simulink model "maglev_sim"  (R2022a)
settings: Solver=VariableStepAuto  StartTime=0.0  StopTime=5  RelTol=1e-3
values from neighbouring files (symbols this model uses):
  A = [ ... (first row only)    [hw3.m]    (also in maglev.m = raw_A - B*K_leader)
  Adj = full(adjacency(Gr))    [hw3.m]    (also in maglev.m = full(adjacency(Gr, 'weighted')))
  B = [0; 1/m1; 0; 0]    [hw3.m]    (also in maglev.m = [0; -9.9453])
  c = 0.7    [hw3.m]    (also in maglev.m = c_values(i))
  C = eye(4)    [hw3.m]    (also in maglev.m = [708.27 0])
  D = diag(in_degrees)    [hw3.m]    (also in maglev.m = 0)
  F = zeros(size(F))    [maglev.m]
  K = inv(R)*(B')*P    [hw3.m]    (also in maglev.m)
  K_leader = acker(raw_A, B, poles)    [maglev.m]
  pins = [1 0 0 0 0 0]    [hw3.m]    (also in maglev.m)
libraries: eeLuenbergerObserver x5
settings Model: Creator=jules  LastModifiedBy=jules
settings DebuggingCC: AllowedUnitSystems=SI,SI (extended)

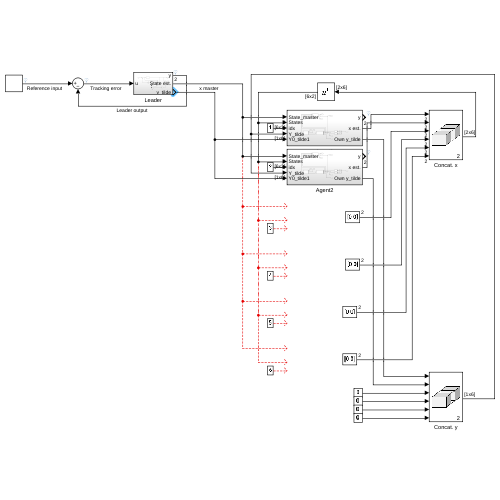
[thumbnail: Simulink's stored preview of the top-level diagram]
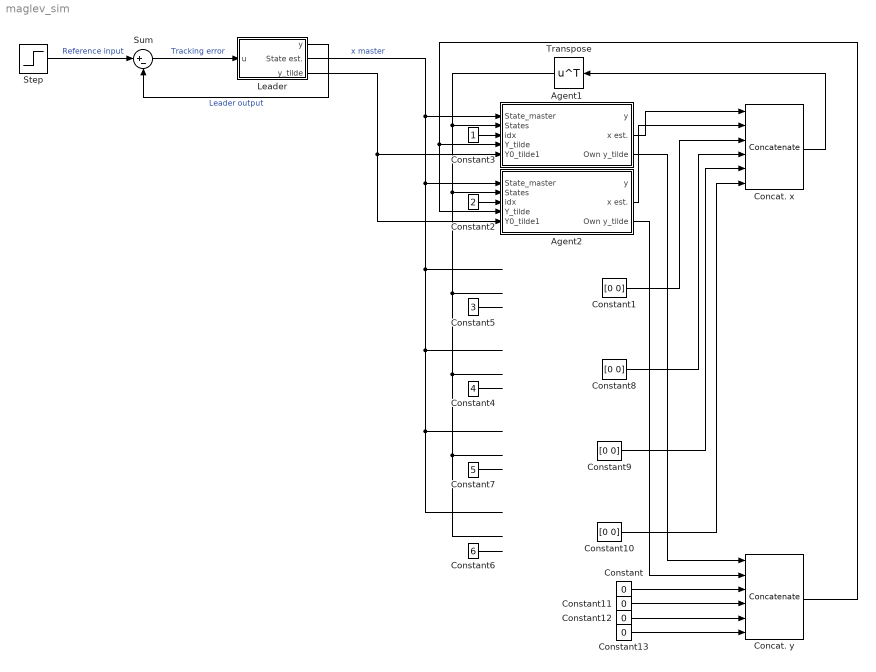
== system maglev_sim ==
  Agent1 : Subsystem
  Agent2 : Subsystem
  Concat. x : Concatenate  NumInputs=6  Mode=Multidimensional array  ConcatenateDimension=2
  Concat. y : Concatenate  NumInputs=6  Mode=Multidimensional array  ConcatenateDimension=2
  Constant{,11..13} (4 alike) : Constant  Value=0
  Constant{1,8..10} (4 alike) : Constant  Value=[0 0]
  Constant2 : Constant  Value=2
  Constant3 : Constant
  Constant4 : Constant  Value=4
  Constant5 : Constant  Value=3
  Constant6 : Constant  Value=6
  Constant7 : Constant  Value=5
  Leader : Subsystem
  Step : Step  SampleTime=0
  Sum : Sum  Inputs=|+-
  Transpose : Math  Operator=transpose
  wires:
  Leader/2(State est.) -> Agent2/1(State_master), Agent1/1(State_master)  "x master"
  Constant3/1 -> Agent1/3(idx)
  Constant4/1 -> ?
  Constant5/1 -> ?
  Constant6/1 -> ?
  Constant7/1 -> ?
  Concat. x/1 -> Transpose/1
  Constant1/1 -> Concat. x/3
  Constant8/1 -> Concat. x/4
  Constant9/1 -> Concat. x/5
  Constant10/1 -> Concat. x/6
  Transpose/1 -> Agent2/2(States), Agent1/2(States)
  Step/1 -> Sum/1  "Reference input"
  Sum/1 -> Leader/1(u)  "Tracking error"
  Leader/1(y) -> Sum/2  "Leader output"
  Agent1/2(x est.) -> Concat. x/1
  Agent1/3(Own y_tilde) -> Concat. y/1
  Constant13/1 -> Concat. y/6
  Constant12/1 -> Concat. y/5
  Constant11/1 -> Concat. y/4
  Constant/1 -> Concat. y/3
  Concat. y/1 -> Agent1/4(Y_tilde), Agent2/4(Y_tilde)
  Constant2/1 -> Agent2/3(idx)
  Agent2/2(x est.) -> Concat. x/2
  Agent2/3(Own y_tilde) -> Concat. y/2
  Leader/3(y_tilde) -> Agent1/5(Y0_tilde1), Agent2/5(Y0_tilde1)

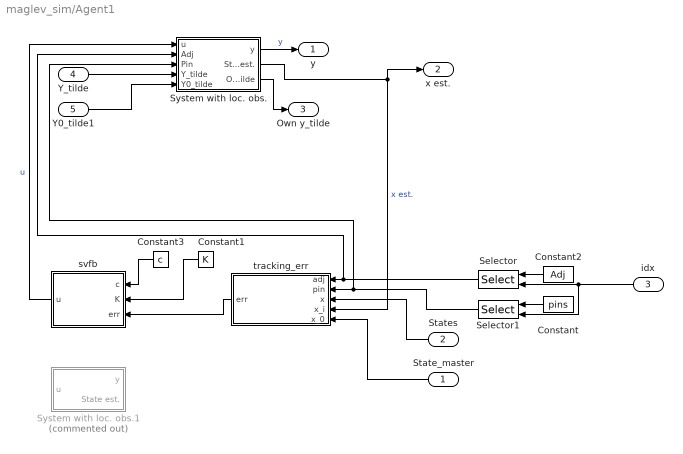
== system maglev_sim/Agent1 ==
  State_master : Inport
  States : Inport  Port=2
  idx : Inport  Port=3
  Y_tilde : Inport  Port=4
  Y0_tilde1 : Inport  Port=5
  Constant : Constant  Value=pins
  Constant1 : Constant  Value=K  VectorParams1D=off
  Constant2 : Constant  Value=Adj  VectorParams1D=off
  Constant3 : Constant  Value=c
  Selector : Selector  NumberOfDimensions=2  InputPortWidth=[6 6]  IndexOptions=Select all,Index vector (port)  Indices=[1 3],1  OutputSizes=1,1
  Selector1 : Selector  InputPortWidth=6  IndexOptions=Index vector (port)  Indices=[1 3]  OutputSizes=1
  System with loc. obs. : Subsystem
  System with loc. obs.1 : Subsystem  Commented=on
  svfb : MATLAB Function  TreatAsAtomicUnit=on
  tracking_err : MATLAB Function  TreatAsAtomicUnit=on
  y : Outport
  x est. : Outport  Port=2
  Own y_tilde : Outport  Port=3
  wires:
  idx/1 -> Selector1/2, Selector/2
  Constant2/1 -> Selector/1
  System with loc. obs./1(y) -> y/1  "y"
  svfb/1(u) -> System with loc. obs./1(u)  "u"
  System with loc. obs./2(State est.) -> tracking_err/4(x_i), x est./1  "x est."
  tracking_err/1(err) -> svfb/3(err)
  Constant/1 -> Selector1/1
  Constant1/1 -> svfb/2(K)
  Constant3/1 -> svfb/1(c)
  States/1 -> tracking_err/3(x)
  State_master/1 -> tracking_err/5(x_0)
  Selector1/1 -> tracking_err/2(pin), System with loc. obs./3(Pin)
  Selector/1 -> System with loc. obs./2(Adj), tracking_err/1(adj)
  System with loc. obs./3(Own y_tilde) -> Own y_tilde/1
  Y_tilde/1 -> System with loc. obs./4(Y_tilde)
  Y0_tilde1/1 -> System with loc. obs./5(Y0_tilde)

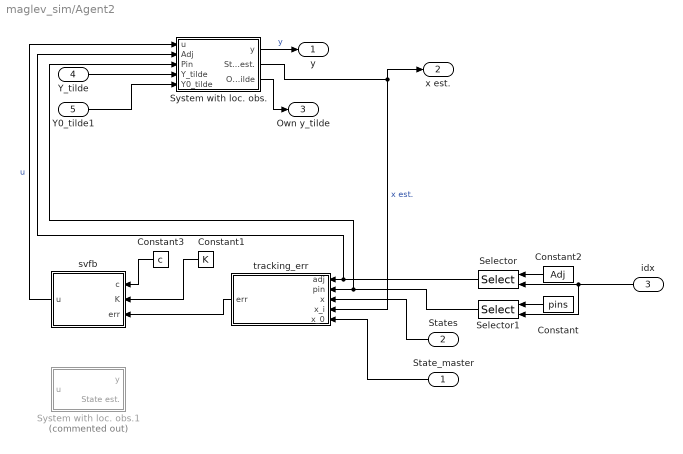
== system maglev_sim/Agent2 ==
  State_master : Inport
  States : Inport  Port=2
  idx : Inport  Port=3
  Y_tilde : Inport  Port=4
  Y0_tilde1 : Inport  Port=5
  Constant : Constant  Value=pins
  Constant1 : Constant  Value=K  VectorParams1D=off
  Constant2 : Constant  Value=Adj  VectorParams1D=off
  Constant3 : Constant  Value=c
  Selector : Selector  NumberOfDimensions=2  InputPortWidth=[6 6]  IndexOptions=Select all,Index vector (port)  Indices=[1 3],1  OutputSizes=1,1
  Selector1 : Selector  InputPortWidth=6  IndexOptions=Index vector (port)  Indices=[1 3]  OutputSizes=1
  System with loc. obs. : Subsystem
  System with loc. obs.1 : Subsystem  Commented=on
  svfb : MATLAB Function  TreatAsAtomicUnit=on
  tracking_err : MATLAB Function  TreatAsAtomicUnit=on
  y : Outport
  x est. : Outport  Port=2
  Own y_tilde : Outport  Port=3
  wires:
  idx/1 -> Selector1/2, Selector/2
  Constant2/1 -> Selector/1
  System with loc. obs./1(y) -> y/1  "y"
  svfb/1(u) -> System with loc. obs./1(u)  "u"
  System with loc. obs./2(State est.) -> tracking_err/4(x_i), x est./1  "x est."
  tracking_err/1(err) -> svfb/3(err)
  Constant/1 -> Selector1/1
  Constant1/1 -> svfb/2(K)
  Constant3/1 -> svfb/1(c)
  States/1 -> tracking_err/3(x)
  State_master/1 -> tracking_err/5(x_0)
  Selector1/1 -> tracking_err/2(pin), System with loc. obs./3(Pin)
  Selector/1 -> System with loc. obs./2(Adj), tracking_err/1(adj)
  System with loc. obs./3(Own y_tilde) -> Own y_tilde/1
  Y_tilde/1 -> System with loc. obs./4(Y_tilde)
  Y0_tilde1/1 -> System with loc. obs./5(Y0_tilde)

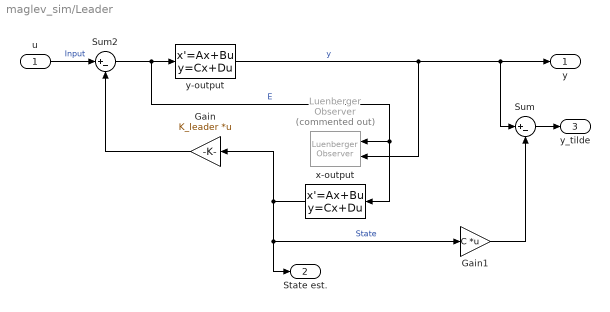
== system maglev_sim/Leader ==
  u : Inport
  Gain : Gain  Gain=K_leader  Multiplication=Matrix(K*u)
  Gain1 : Gain  Gain=C  Multiplication=Matrix(K*u)
  Luenberger Observer : eeLuenbergerObserver/Luenberger Observer  Commented=on  StateSpaceType=Continuous-time  Ad=A  Bd=1  Cd=1  Dd=1  A=A  B=B  C=C  D=[0]  ObserverDesign=Desired eigenvalues  Ld=1  DesiredEigenvalues=[-10 -20]  x0=[0 0]  Tsd=0.1  Ts=0.1
      settings: SourceProductBaseCode=PS
  Sum : Sum  Inputs=|+-
  Sum2 : Sum  Inputs=|+-
  x-output : StateSpace  A=A  B=B  C=eye(2)  D=[0; 0]  InitialCondition=0
  y-output : StateSpace  A=A  B=B  C=C  D=D  InitialCondition=0
  y : Outport
  State est. : Outport  Port=2
  y_tilde : Outport  Port=3
  wires:
  Gain/1 -> Sum2/2
  y-output/1 -> Luenberger Observer/2, Sum/1, y/1  "y"
  u/1 -> Sum2/1  "Input"
  Sum2/1 -> Luenberger Observer/1, x-output/1, y-output/1  "E"
  x-output/1 -> Gain1/1, State est./1, Gain/1  "State"
  Gain1/1 -> Sum/2
  Sum/1 -> y_tilde/1

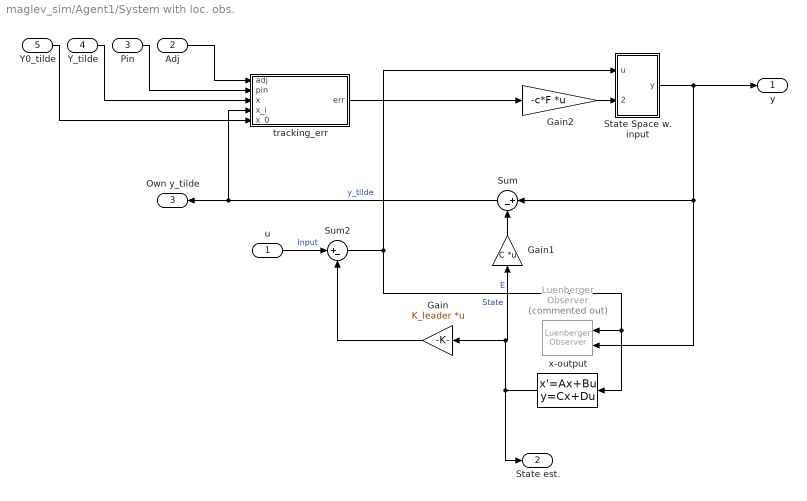
== system maglev_sim/Agent1/System with loc. obs. ==
  u : Inport
  Adj : Inport  Port=2
  Pin : Inport  Port=3
  Y_tilde : Inport  Port=4
  Y0_tilde : Inport  Port=5
  Gain : Gain  Gain=K_leader  Multiplication=Matrix(K*u)
  Gain1 : Gain  Gain=C  Multiplication=Matrix(K*u)
  Gain2 : Gain  Gain=-c*F  Multiplication=Matrix(K*u)
  Luenberger Observer : eeLuenbergerObserver/Luenberger Observer  Commented=on  StateSpaceType=Continuous-time  Ad=A  Bd=1  Cd=1  Dd=1  A=A  B=B  C=C  D=[0]  ObserverDesign=Desired eigenvalues  Ld=1  DesiredEigenvalues=[-10 -20]  x0=[0 0]  Tsd=0.1  Ts=0.1
      settings: SourceProductBaseCode=PS
  State Space w. input : Subsystem
  Sum : Sum  Inputs=|+-
  Sum2 : Sum  Inputs=|+-
  tracking_err : MATLAB Function  TreatAsAtomicUnit=on
  x-output : StateSpace  A=A  B=B  C=eye(2)  D=[0; 0]  InitialCondition=0
  y : Outport
  State est. : Outport  Port=2
  Own y_tilde : Outport  Port=3
  wires:
  Gain/1 -> Sum2/2
  u/1 -> Sum2/1  "Input"
  Sum2/1 -> State Space w. input/1(u), Luenberger Observer/1, x-output/1  "E"
  x-output/1 -> State est./1, Gain1/1, Gain/1  "State"
  State Space w. input/1(y) -> Sum/1, Luenberger Observer/2, y/1
  Gain2/1 -> State Space w. input/2(extra)
  tracking_err/1(err) -> Gain2/1
  Adj/1 -> tracking_err/1(adj)
  Pin/1 -> tracking_err/2(pin)
  Y_tilde/1 -> tracking_err/3(x)
  Y0_tilde/1 -> tracking_err/5(x_0)
  Gain1/1 -> Sum/2
  Sum/1 -> Own y_tilde/1, tracking_err/4(x_i)  "y_tilde"

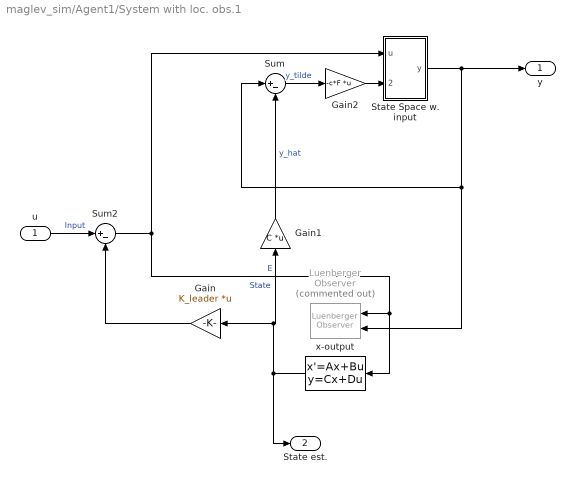
== system maglev_sim/Agent1/System with loc. obs.1 ==
  u : Inport
  Gain : Gain  Gain=K_leader  Multiplication=Matrix(K*u)
  Gain1 : Gain  Gain=C  Multiplication=Matrix(K*u)
  Gain2 : Gain  Gain=-c*F  Multiplication=Matrix(K*u)
  Luenberger Observer : eeLuenbergerObserver/Luenberger Observer  Commented=on  StateSpaceType=Continuous-time  Ad=A  Bd=1  Cd=1  Dd=1  A=A  B=B  C=C  D=[0]  ObserverDesign=Desired eigenvalues  Ld=1  DesiredEigenvalues=[-10 -20]  x0=[0 0]  Tsd=0.1  Ts=0.1
      settings: SourceProductBaseCode=PS
  State Space w. input : Subsystem
  Sum : Sum  Inputs=|+-
  Sum2 : Sum  Inputs=|+-
  x-output : StateSpace  A=A  B=B  C=eye(2)  D=[0; 0]  InitialCondition=0
  y : Outport
  State est. : Outport  Port=2
  wires:
  Gain/1 -> Sum2/2
  u/1 -> Sum2/1  "Input"
  Sum2/1 -> State Space w. input/1(u), Luenberger Observer/1, x-output/1  "E"
  x-output/1 -> State est./1, Gain1/1, Gain/1  "State"
  State Space w. input/1(y) -> Sum/1, Luenberger Observer/2, y/1
  Sum/1 -> Gain2/1  "y_tilde"
  Gain1/1 -> Sum/2  "y_hat"
  Gain2/1 -> State Space w. input/2(extra)

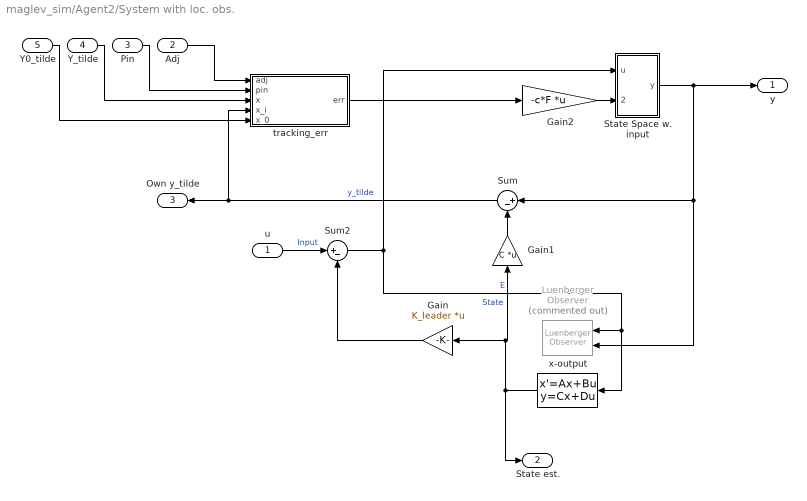
== system maglev_sim/Agent2/System with loc. obs. ==
  u : Inport
  Adj : Inport  Port=2
  Pin : Inport  Port=3
  Y_tilde : Inport  Port=4
  Y0_tilde : Inport  Port=5
  Gain : Gain  Gain=K_leader  Multiplication=Matrix(K*u)
  Gain1 : Gain  Gain=C  Multiplication=Matrix(K*u)
  Gain2 : Gain  Gain=-c*F  Multiplication=Matrix(K*u)
  Luenberger Observer : eeLuenbergerObserver/Luenberger Observer  Commented=on  StateSpaceType=Continuous-time  Ad=A  Bd=1  Cd=1  Dd=1  A=A  B=B  C=C  D=[0]  ObserverDesign=Desired eigenvalues  Ld=1  DesiredEigenvalues=[-10 -20]  x0=[0 0]  Tsd=0.1  Ts=0.1
      settings: SourceProductBaseCode=PS
  State Space w. input : Subsystem
  Sum : Sum  Inputs=|+-
  Sum2 : Sum  Inputs=|+-
  tracking_err : MATLAB Function  TreatAsAtomicUnit=on
  x-output : StateSpace  A=A  B=B  C=eye(2)  D=[0; 0]  InitialCondition=0
  y : Outport
  State est. : Outport  Port=2
  Own y_tilde : Outport  Port=3
  wires:
  Gain/1 -> Sum2/2
  u/1 -> Sum2/1  "Input"
  Sum2/1 -> State Space w. input/1(u), Luenberger Observer/1, x-output/1  "E"
  x-output/1 -> State est./1, Gain1/1, Gain/1  "State"
  State Space w. input/1(y) -> Sum/1, Luenberger Observer/2, y/1
  Gain2/1 -> State Space w. input/2(extra)
  tracking_err/1(err) -> Gain2/1
  Adj/1 -> tracking_err/1(adj)
  Pin/1 -> tracking_err/2(pin)
  Y_tilde/1 -> tracking_err/3(x)
  Y0_tilde/1 -> tracking_err/5(x_0)
  Gain1/1 -> Sum/2
  Sum/1 -> Own y_tilde/1, tracking_err/4(x_i)  "y_tilde"

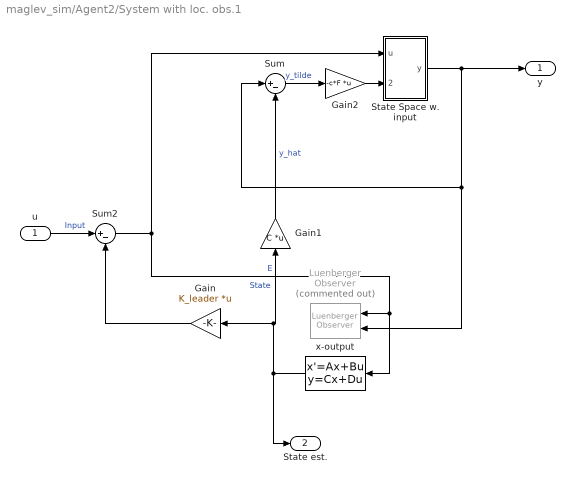
== system maglev_sim/Agent2/System with loc. obs.1 ==
  u : Inport
  Gain : Gain  Gain=K_leader  Multiplication=Matrix(K*u)
  Gain1 : Gain  Gain=C  Multiplication=Matrix(K*u)
  Gain2 : Gain  Gain=-c*F  Multiplication=Matrix(K*u)
  Luenberger Observer : eeLuenbergerObserver/Luenberger Observer  Commented=on  StateSpaceType=Continuous-time  Ad=A  Bd=1  Cd=1  Dd=1  A=A  B=B  C=C  D=[0]  ObserverDesign=Desired eigenvalues  Ld=1  DesiredEigenvalues=[-10 -20]  x0=[0 0]  Tsd=0.1  Ts=0.1
      settings: SourceProductBaseCode=PS
  State Space w. input : Subsystem
  Sum : Sum  Inputs=|+-
  Sum2 : Sum  Inputs=|+-
  x-output : StateSpace  A=A  B=B  C=eye(2)  D=[0; 0]  InitialCondition=0
  y : Outport
  State est. : Outport  Port=2
  wires:
  Gain/1 -> Sum2/2
  u/1 -> Sum2/1  "Input"
  Sum2/1 -> State Space w. input/1(u), Luenberger Observer/1, x-output/1  "E"
  x-output/1 -> State est./1, Gain1/1, Gain/1  "State"
  State Space w. input/1(y) -> Sum/1, Luenberger Observer/2, y/1
  Sum/1 -> Gain2/1  "y_tilde"
  Gain1/1 -> Sum/2  "y_hat"
  Gain2/1 -> State Space w. input/2(extra)

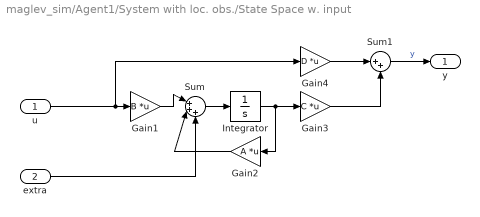
== system maglev_sim/Agent1/System with loc. obs./State Space w. input ==
  u : Inport
  extra : Inport  Port=2
  Gain1 : Gain  Gain=B  Multiplication=Matrix(K*u)
  Gain2 : Gain  Gain=A  Multiplication=Matrix(K*u)
  Gain3 : Gain  Gain=C  Multiplication=Matrix(K*u)
  Gain4 : Gain  Gain=D  Multiplication=Matrix(K*u)
  Integrator : Integrator
  Sum : Sum  Inputs=|+++
  Sum1 : Sum  Inputs=|++
  y : Outport
  wires:
  Gain3/1 -> Sum1/2
  Gain2/1 -> Sum/2
  Gain1/1 -> Sum/1
  u/1 -> Gain4/1, Gain1/1
  Sum/1 -> Integrator/1
  Gain4/1 -> Sum1/1
  Sum1/1 -> y/1  "y"
  Integrator/1 -> Gain3/1, Gain2/1
  extra/1 -> Sum/3

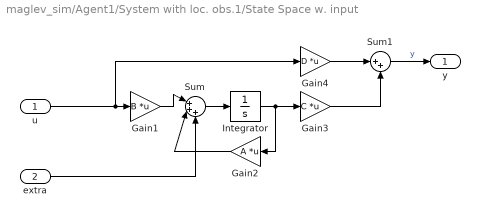
== system maglev_sim/Agent1/System with loc. obs.1/State Space w. input ==
  u : Inport
  extra : Inport  Port=2
  Gain1 : Gain  Gain=B  Multiplication=Matrix(K*u)
  Gain2 : Gain  Gain=A  Multiplication=Matrix(K*u)
  Gain3 : Gain  Gain=C  Multiplication=Matrix(K*u)
  Gain4 : Gain  Gain=D  Multiplication=Matrix(K*u)
  Integrator : Integrator
  Sum : Sum  Inputs=|+++
  Sum1 : Sum  Inputs=|++
  y : Outport
  wires:
  Gain3/1 -> Sum1/2
  Gain2/1 -> Sum/2
  Gain1/1 -> Sum/1
  u/1 -> Gain4/1, Gain1/1
  Sum/1 -> Integrator/1
  Gain4/1 -> Sum1/1
  Sum1/1 -> y/1  "y"
  Integrator/1 -> Gain3/1, Gain2/1
  extra/1 -> Sum/3

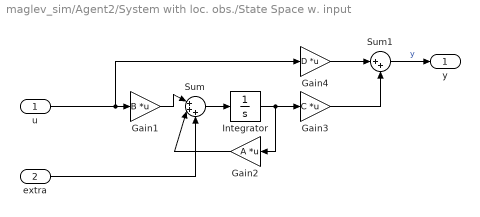
== system maglev_sim/Agent2/System with loc. obs./State Space w. input ==
  u : Inport
  extra : Inport  Port=2
  Gain1 : Gain  Gain=B  Multiplication=Matrix(K*u)
  Gain2 : Gain  Gain=A  Multiplication=Matrix(K*u)
  Gain3 : Gain  Gain=C  Multiplication=Matrix(K*u)
  Gain4 : Gain  Gain=D  Multiplication=Matrix(K*u)
  Integrator : Integrator
  Sum : Sum  Inputs=|+++
  Sum1 : Sum  Inputs=|++
  y : Outport
  wires:
  Gain3/1 -> Sum1/2
  Gain2/1 -> Sum/2
  Gain1/1 -> Sum/1
  u/1 -> Gain4/1, Gain1/1
  Sum/1 -> Integrator/1
  Gain4/1 -> Sum1/1
  Sum1/1 -> y/1  "y"
  Integrator/1 -> Gain3/1, Gain2/1
  extra/1 -> Sum/3

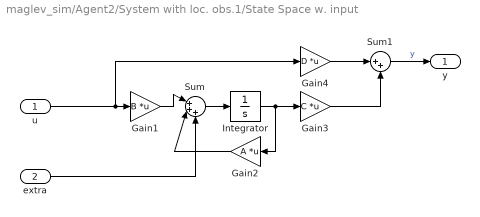
== system maglev_sim/Agent2/System with loc. obs.1/State Space w. input ==
  u : Inport
  extra : Inport  Port=2
  Gain1 : Gain  Gain=B  Multiplication=Matrix(K*u)
  Gain2 : Gain  Gain=A  Multiplication=Matrix(K*u)
  Gain3 : Gain  Gain=C  Multiplication=Matrix(K*u)
  Gain4 : Gain  Gain=D  Multiplication=Matrix(K*u)
  Integrator : Integrator
  Sum : Sum  Inputs=|+++
  Sum1 : Sum  Inputs=|++
  y : Outport
  wires:
  Gain3/1 -> Sum1/2
  Gain2/1 -> Sum/2
  Gain1/1 -> Sum/1
  u/1 -> Gain4/1, Gain1/1
  Sum/1 -> Integrator/1
  Gain4/1 -> Sum1/1
  Sum1/1 -> y/1  "y"
  Integrator/1 -> Gain3/1, Gain2/1
  extra/1 -> Sum/3

== matlab function maglev_sim/Agent1/svfb ==
  data: c input; K input; u output; err input
function u = svfb(c, K, err)
u = 0;
u = u + (c * K * err)';

== matlab function maglev_sim/Agent1/tracking_err ==
  data: adj input; pin input; x input; x_i input; x_0 input; err output
function err = tracking_err(adj, pin, x, x_i, x_0)
err = zeros([2 1]);
err = err + pin * (x_0 - x_i);
for j = 1:6
    err = err + adj(j) * (x(j) - x_i);
end

== matlab function maglev_sim/Agent2/System with loc. obs./tracking_err ==
  data: adj input; pin input; x input; x_i input; x_0 input; err output
function err = tracking_err(adj, pin, x, x_i, x_0)
err = 0;
err = err + pin * (x_0 - x_i);
for j = 1:6
    err = err + adj(j) * (x(j) - x_i);
end

== matlab function maglev_sim/Agent2/svfb ==
  data: c input; K input; u output; err input
function u = svfb(c, K, err)
u = 0;
u = u + (c * K * err)';

== matlab function maglev_sim/Agent1/System with loc. obs./tracking_err ==
  data: adj input; pin input; x input; x_i input; x_0 input; err output
function err = tracking_err(adj, pin, x, x_i, x_0)
err = 0;
err = err + pin * (x_0 - x_i);
for j = 1:6
    err = err + adj(j) * (x(j) - x_i);
end

== matlab function maglev_sim/Agent2/tracking_err ==
  data: adj input; pin input; x input; x_i input; x_0 input; err output
function err = tracking_err(adj, pin, x, x_i, x_0)
err = zeros([2 1]);
err = err + pin * (x_0 - x_i);
for j = 1:6
    err = err + adj(j) * (x(j) - x_i);
end
